simulink model "pathPredict"  (R2015b)
settings: Solver=VariableStepAuto  StartTime=0.0  StopTime=10.0  RelTol=1e-3
settings Model: Creator=tcyu  LastModifiedBy=tcyu

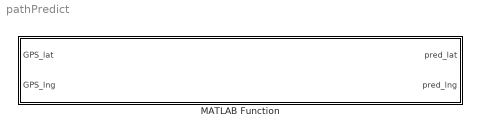
== system pathPredict ==
  MATLAB Function : MATLAB Function  TreatAsAtomicUnit=on

== matlab function pathPredict/MATLAB Function ==
  data: GPS_lat input; pred_lat output; GPS_lng input; pred_lng output
function [pred_lat,pred_lng] = pathPredict(GPS_lat,GPS_lng)
prediction = vehiclePathPredObj.pathPredict(GPS_lat,GPS_lng);
pred_lat = prediction(:,1);
pred_lng = prediction(:,2);
end
